simulink model "Turbine_TestBed"  (R2015a)
settings: Solver=FixedStepDiscrete  StartTime=0.0  StopTime=1  FixedStep=1  RelTol=1e-3
undefined symbols (not defined in the file): MWS, stripchar_TMATS
libraries: Lib_Turbo_Turbine_TMATS x1
settings Model: Creator=jwchapm2  LastModifiedBy=jwchapm2
settings OptimizationCC: ExpressionDepthLimit=2147483647
settings DebuggingCC: UnderspecifiedInitializationDetection=Classic  MergeDetectMultiDrivingBlocksExec=none  SolverPrmCheckMsg=warning  StateNameClashWarn=warning

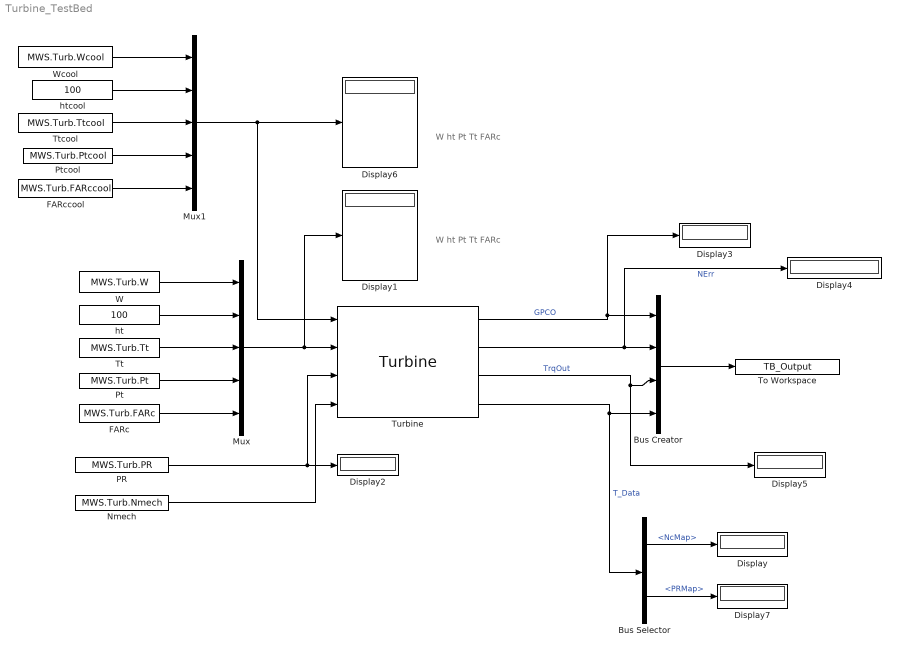
== system Turbine_TestBed ==
  note: W
      | ht
      | Pt
      | Tt
      | FARc
  note: W
      | ht
      | Pt
      | Tt
      | FARc
  Bus Selector : BusSelector  OutputSignals=NcMap,PRMap
  Bus Creator : BusCreator
  Display{,1..7} (8 alike) : Display
  FARc : Constant  Value=MWS.Turb.FARc
  FARccool : Constant  Value=MWS.Turb.FARccool
  Mux : Mux  Inputs=5
  Mux1 : Mux  Inputs=5
  Nmech : Constant  Value=MWS.Turb.Nmech
  PR : Constant  Value=MWS.Turb.PR
  Pt : Constant  Value=MWS.Turb.Pt
  Ptcool : Constant  Value=MWS.Turb.Ptcool
  To Workspace : ToWorkspace  VariableName=TB_Output  SampleTime=-1
  Tt : Constant  Value=MWS.Turb.Tt
  Ttcool : Constant  Value=MWS.Turb.Ttcool
  Turbine : Lib_Turbo_Turbine_TMATS/Turbine  X_T_Map_PRVec_M=MWS.Turb.PRVec  Y_T_Map_NcVec_M=MWS.Turb.NcVec  T_T_Map_WcArray_M=MWS.Turb.WcArray  T_T_Map_EffArray_M=MWS.Turb.EffArray  s_T_Nc_M=MWS.Turb.s_Nc  s_T_Wc_M=MWS.Turb.s_Wc  s_T_PR_M=MWS.Turb.s_PR  s_T_Eff_M=MWS.Turb.s_eff  ConfigNPSS_M=0  Scale_M=none  CFlwEn_M=on  T_CoolFlwPos_M=MWS.Turb.CF  iDesign_M=2  NcDes_M=100  EffDes_M=0.9328  PRDes_M=5  NDes_M=10000  FVar_M=strcat('iDes_',stripchar_TMATS(gcb),'.bin')  BlkNm_M=double(gcb)  HP_M=off
  W : Constant  Value=MWS.Turb.W
  Wcool : Constant  Value=MWS.Turb.Wcool
  ht : Constant  Value=100
  htcool : Constant  Value=100
  wires:
  PR/1 -> Turbine/3, Display2/1
  W/1 -> Mux/1
  FARc/1 -> Mux/5
  Tt/1 -> Mux/3
  Pt/1 -> Mux/4
  Mux/1 -> Display1/1, Turbine/2
  Turbine/1 -> Bus Creator/1, Display3/1  "GPCO"
  Turbine/2 -> Bus Creator/2, Display4/1  "NErr"
  Turbine/3 -> Bus Creator/3, Display5/1  "TrqOut"
  Turbine/4 -> Bus Selector/1, Bus Creator/4  "T_Data"
  Bus Creator/1 -> To Workspace/1
  ht/1 -> Mux/2
  Nmech/1 -> Turbine/4
  Wcool/1 -> Mux1/1
  FARccool/1 -> Mux1/5
  Ttcool/1 -> Mux1/3
  Ptcool/1 -> Mux1/4
  Mux1/1 -> Display6/1, Turbine/1
  htcool/1 -> Mux1/2
  Bus Selector/1 -> Display/1  "<NcMap>"
  Bus Selector/2 -> Display7/1  "<PRMap>"
